simulink model "model_gyro_sim"  (R2021b)
settings: Solver=FixedStepAuto  StartTime=0.0  StopTime=time  FixedStep=1/(fs)  RelTol=1e-3
values from neighbouring files (symbols this model uses):
  arw_std = arw_in*sqrt(fc)    [main.m]
  bias_in = bias_in/3600    (= 4.72222222222e-07)    [main.m]
  fs = 100    [main.m]
  w_ie_down = w_ie_down/3600    [main.m]
settings Model: Creator=User  LastModifiedBy=Stinky

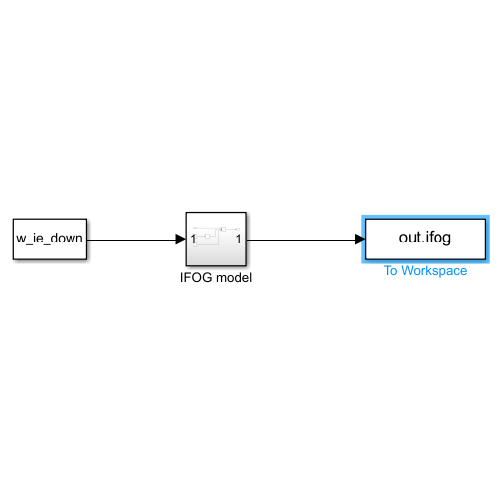
[thumbnail: Simulink's stored preview of the top-level diagram]
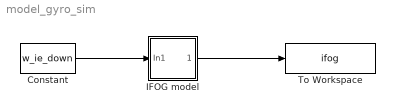
== system model_gyro_sim ==
  Constant : Constant  Value=w_ie_down
  IFOG model : Subsystem
  To Workspace : ToWorkspace  VariableName=ifog  SaveFormat=Timeseries  SampleTime=-1
  wires:
  Constant/1 -> IFOG model/1(In1)
  IFOG model/1(Out1) -> To Workspace/1

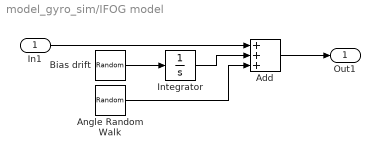
== system model_gyro_sim/IFOG model ==
  In1 : Inport
  Add : Sum  Inputs=+++
  Angle Random Walk : RandomNumber  Variance=arw_std^2  SampleTime=1/fs
  Bias drift : RandomNumber  Variance=bias_in^2  SampleTime=1/fs
  Integrator : Integrator
  Out1 : Outport
  wires:
  In1/1 -> Add/1
  Add/1 -> Out1/1
  Angle Random Walk/1 -> Add/3
  Bias drift/1 -> Integrator/1
  Integrator/1 -> Add/2
